simulink model "TestWeak_xD"  (R2022a)
settings: Solver=VariableStepAuto  StartTime=0.0  StopTime=inf  RelTol=1e-3
undefined symbols (not defined in the file or in its folder): DiscIntNeverNeededParam
libraries: simulink x2, rllib x2
settings Model: Creator=yifei  LastModifiedBy=yifei

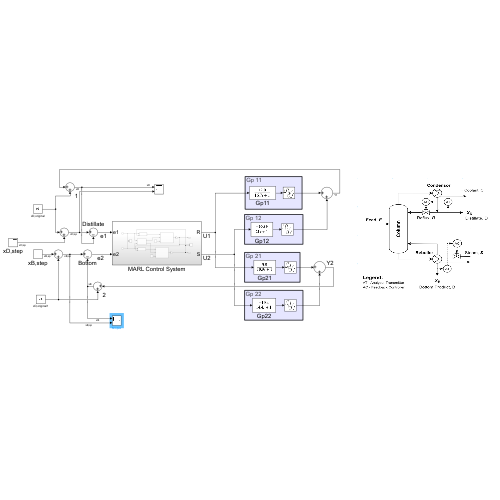
[thumbnail: Simulink's stored preview of the top-level diagram]
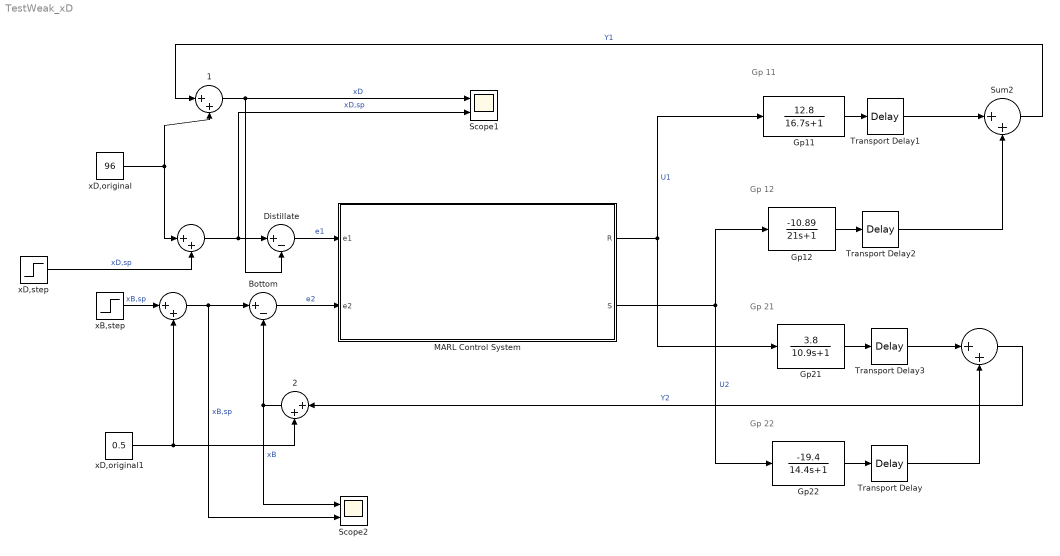
== system TestWeak_xD ==
  note: Gp 11
  note: Gp 22
  note: Gp 12
  note: Gp 21
  " " : Sum  Inputs=|++
  "     " : Sum  Inputs=|++
  "        " : Sum  Inputs=|++
  "        1" : Sum  Inputs=|++
  "        2" : Sum  Inputs=|++
  Bottom : Sum  Inputs=|+-
  Distillate : Sum  Inputs=|+-
  Gp11 : TransferFcn  Numerator=[12.8]  Denominator=[16.7 1]
  Gp12 : TransferFcn  Numerator=[-10.89]  Denominator=[21 1]
  Gp21 : TransferFcn  Numerator=[3.8]  Denominator=[10.9 1]
  Gp22 : TransferFcn  Numerator=[-19.4]  Denominator=[14.4 1]
  MARL Control System : Subsystem
  Scope1 : Scope  NumInputPorts=2
  Scope2 : Scope  NumInputPorts=2
  Sum2 : Sum  Inputs=|++
  Transport Delay : TransportDelay  DelayTime=3
  Transport Delay1 : TransportDelay
  Transport Delay2 : TransportDelay  DelayTime=3
  Transport Delay3 : TransportDelay  DelayTime=2
  xB,step : Step  Time=2  After=0  SampleTime=0  ZeroCross=off
  xD,original : Constant  Value=96
  xD,original1 : Constant  Value=0.5
  xD,step : Step  Time=2  SampleTime=0  ZeroCross=off
  wires:
  Gp21/1 -> Transport Delay3/1
  MARL Control System/1(R) -> Gp21/1, Gp11/1  "U1"
  Gp12/1 -> Transport Delay2/1
  Gp22/1 -> Transport Delay/1
  Gp11/1 -> Transport Delay1/1
  Bottom/1 -> MARL Control System/2(e2)  "e2"
  Distillate/1 -> MARL Control System/1(e1)  "e1"
  MARL Control System/2(S) -> Gp22/1, Gp12/1  "U2"
  Transport Delay2/1 -> Sum2/2
  " "/1 -> "        2"/1  "Y2"
  Transport Delay1/1 -> Sum2/1
  Transport Delay3/1 -> " "/1
  Transport Delay/1 -> " "/2
  xD,original1/1 -> "        2"/2, "     "/2
  "        "/1 -> Scope1/2, Distillate/1  "xD,sp"
  xD,step/1 -> "        "/2  "xD,sp"
  xD,original/1 -> "        1"/2, "        "/1
  xB,step/1 -> "     "/1  "xB,sp"
  Sum2/1 -> "        1"/1  "Y1"
  "        1"/1 -> Distillate/2, Scope1/1  "xD"
  "        2"/1 -> Scope2/1, Bottom/2  "xB"
  "     "/1 -> Scope2/2, Bottom/1  "xB,sp"

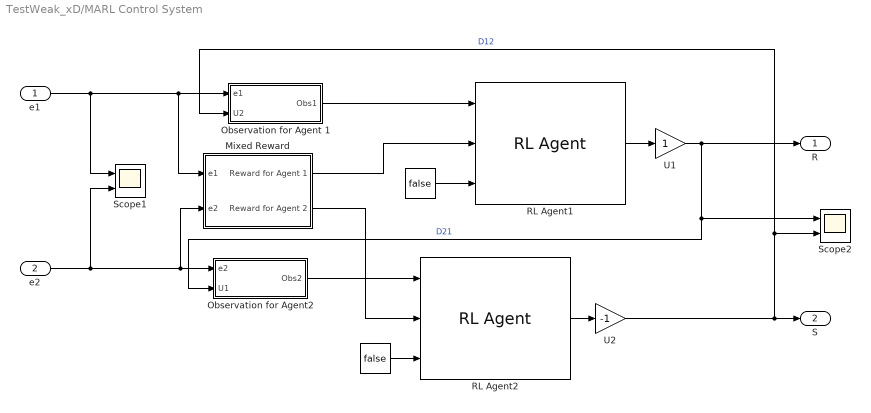
== system TestWeak_xD/MARL Control System ==
  e1 : Inport
  e2 : Inport  Port=2
  "       " : Constant  Value=false
  "            " : Constant  Value=false
  Mixed Reward : Subsystem
  Observation for Agent 1 : Subsystem
  Observation for Agent2 : Subsystem
  RL Agent1 : rllib/RL Agent  Agent=agentObj1  ExternalActionAsInput=off  ProvideLastAction=off  ProvideCumRwd=off  TreatAsDirectFeedthrough=on  UseStrictObservationDataTypes=off
  RL Agent2 : rllib/RL Agent  Agent=agentObj2  ExternalActionAsInput=off  ProvideLastAction=off  ProvideCumRwd=off  TreatAsDirectFeedthrough=on  UseStrictObservationDataTypes=off
  Scope1 : Scope  NumInputPorts=2
  Scope2 : Scope  NumInputPorts=2
  U1 : Gain
  U2 : Gain  Gain=-1
  R : Outport
  S : Outport  Port=2
  wires:
  "       "/1 -> RL Agent2/3
  "            "/1 -> RL Agent1/3
  RL Agent1/1 -> U1/1
  RL Agent2/1 -> U2/1
  Observation for Agent 1/1(Obs1) -> RL Agent1/1
  Observation for Agent2/1(Obs2) -> RL Agent2/1
  e1/1 -> Scope1/1, Mixed Reward/1("e1 "), Observation for Agent 1/1(e1)
  e2/1 -> Scope1/2, Observation for Agent2/1(e2), Mixed Reward/2(e2)
  U2/1 -> S/1, Observation for Agent 1/2(U2), Scope2/2  "D12"
  U1/1 -> R/1, Scope2/1, Observation for Agent2/2(U1)  "D21"
  Mixed Reward/2(Reward for Agent 2) -> RL Agent2/2
  Mixed Reward/1(Reward for Agent 1) -> RL Agent1/2

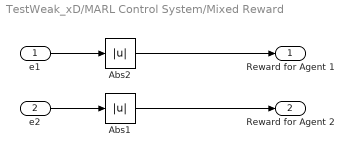
== system TestWeak_xD/MARL Control System/Mixed Reward ==
  "e1 " : Inport
  e2 : Inport  Port=2
  Abs1 : Abs  SaturateOnIntegerOverflow=off
  Abs2 : Abs  SaturateOnIntegerOverflow=off
  Reward for Agent 1 : Outport
  Reward for Agent 2 : Outport  Port=2
  wires:
  e2/1 -> Abs1/1
  "e1 "/1 -> Abs2/1
  Abs2/1 -> Reward for Agent 1/1
  Abs1/1 -> Reward for Agent 2/1

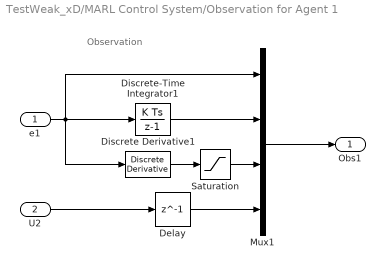
== system TestWeak_xD/MARL Control System/Observation for Agent 1 ==
  note: Observation
  e1 : Inport
  U2 : Inport  Port=2
  Delay : Delay  DelayLength=1  InitialCondition=0
  Discrete Derivative1 : simulink/Discrete/Discrete Derivative  gainval=1  ICPrevScaledInput=0.0  OutMin=[]  OutMax=[]  OutDataType=fixdt(1, 16)  OutScaling=2^-10  DoSatur=off
  Discrete-Time Integrator1 : DiscreteIntegrator  gainval=0.2  SampleTime=-1  ICPrevOutput=DiscIntNeverNeededParam  ICPrevScaledInput=DiscIntNeverNeededParam
  Mux1 : Mux
  Saturation : Saturate  LinearizeAsGain=off  ZeroCross=off
  Obs1 : Outport
  wires:
  Discrete-Time Integrator1/1 -> Mux1/2
  Mux1/1 -> Obs1/1
  Discrete Derivative1/1 -> Saturation/1
  e1/1 -> Mux1/1, Discrete Derivative1/1, Discrete-Time Integrator1/1
  Saturation/1 -> Mux1/3
  Delay/1 -> Mux1/4
  U2/1 -> Delay/1

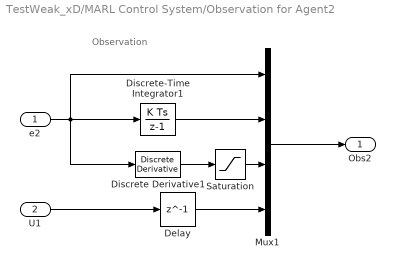
== system TestWeak_xD/MARL Control System/Observation for Agent2 ==
  note: Observation
  e2 : Inport
  U1 : Inport  Port=2
  Delay : Delay  DelayLength=1  InitialCondition=0
  Discrete Derivative1 : simulink/Discrete/Discrete Derivative  gainval=1.5  ICPrevScaledInput=0.0  OutMin=[]  OutMax=[]  OutDataType=fixdt(1, 16)  OutScaling=2^-10  DoSatur=off
  Discrete-Time Integrator1 : DiscreteIntegrator  gainval=1/8  SampleTime=-1  ICPrevOutput=DiscIntNeverNeededParam  ICPrevScaledInput=DiscIntNeverNeededParam
  Mux1 : Mux
  Saturation : Saturate  LinearizeAsGain=off  ZeroCross=off
  Obs2 : Outport
  wires:
  Saturation/1 -> Mux1/3
  Discrete Derivative1/1 -> Saturation/1
  e2/1 -> Mux1/1, Discrete Derivative1/1, Discrete-Time Integrator1/1
  Mux1/1 -> Obs2/1
  Discrete-Time Integrator1/1 -> Mux1/2
  Delay/1 -> Mux1/4
  U1/1 -> Delay/1
